simulink model "coeff_bank_simple_test"  (R2021b)
settings: Solver=FixedStepDiscrete  StartTime=0.0  StopTime=stop_time  RelTol=1e-3
values from neighbouring files (symbols this model uses):
  coeff_bitwidth = ul_filter_attribs.coeff_bitwidth    [coeff_bank_simple_testground.m]
  coeff_complex = ul_filter_attribs.complex    [coeff_bank_simple_testground.m]
  coeff_num = ul_filter_attribs.coeff_num    [coeff_bank_simple_testground.m]
libraries: dspsrcs4 x4
settings Model: DataTypeOverride=Off  Creator=torha  LastModifiedBy=torha
settings SolverCC: AlgebraicLoopSolver=TrustRegion
settings OptimizationCC: BlockReduction=off  ConditionallyExecuteInputs=off  DefaultParameterBehavior=Inlined  InheritOutputTypeSmallerThanSingle=on
settings DebuggingCC: AlgebraicLoopMsg=error  SingleTaskRateTransMsg=error  SFMachineParentedDataDiag=warning
settings HardwareCC: ProdBitPerPointer=32  ProdBitPerSizeT=32  ProdBitPerPtrDiffT=32  ProdLargestAtomicFloat=None  ProdIntDivRoundTo=Undefined  ProdEndianess=Unspecified  ProdWordSize=32  ProdHWDeviceType=ASIC/FPGA->ASIC/FPGA  TargetBitPerPointer=64  TargetBitPerSizeT=64  TargetBitPerPtrDiffT=64  TargetLongLongMode=on  TargetIntDivRoundTo=Zero  TargetEndianess=LittleEndian  TargetWordSize=64  TargetHWDeviceType=Custom Processor->MATLAB Host Computer  ProdEqTarget=off

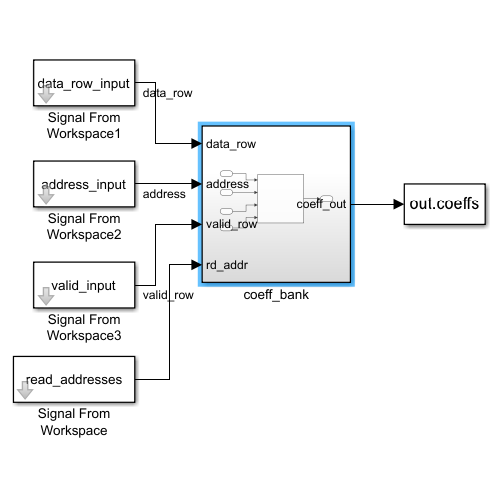
[thumbnail: Simulink's stored preview of the top-level diagram]
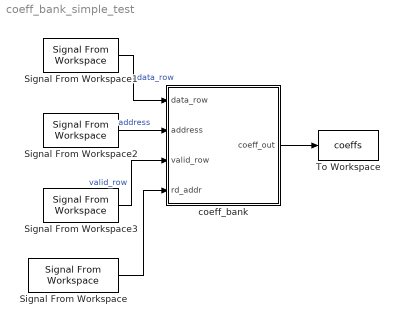
== system coeff_bank_simple_test ==
  Signal From Workspace : dspsrcs4/Signal From Workspace  X=read_addresses  Ts=1  nsamps=1  OutputAfterFinalValue=Setting to zero  ignoreOrWarnInputAndFrameLengths=off  OutputFrames=off
  Signal From Workspace1 : dspsrcs4/Signal From Workspace  X=data_row_input  Ts=1  nsamps=1  OutputAfterFinalValue=Setting to zero  ignoreOrWarnInputAndFrameLengths=off  OutputFrames=off
  Signal From Workspace2 : dspsrcs4/Signal From Workspace  X=address_input  Ts=1  nsamps=1  OutputAfterFinalValue=Setting to zero  ignoreOrWarnInputAndFrameLengths=off  OutputFrames=off
  Signal From Workspace3 : dspsrcs4/Signal From Workspace  X=valid_input  Ts=1  nsamps=1  OutputAfterFinalValue=Setting to zero  ignoreOrWarnInputAndFrameLengths=off  OutputFrames=off
  To Workspace : ToWorkspace  VariableName=coeffs  SampleTime=-1
      settings: Save2DSignal=2-D array (concatenate along first dimension)
  coeff_bank : Subsystem
  wires:
  Signal From Workspace/1 -> coeff_bank/4(rd_addr)
  coeff_bank/1(coeff_out) -> To Workspace/1
  Signal From Workspace2/1 -> coeff_bank/2(address)  "address"
  Signal From Workspace3/1 -> coeff_bank/3(valid_row)  "valid_row"
  Signal From Workspace1/1 -> coeff_bank/1(data_row)  "data_row"

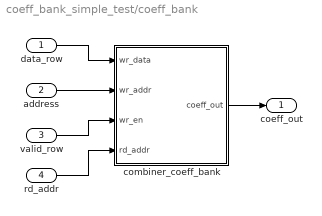
== system coeff_bank_simple_test/coeff_bank ==
  data_row : Inport
  address : Inport  Port=2
  valid_row : Inport  Port=3
  rd_addr : Inport  Port=4
  combiner_coeff_bank : Subsystem  Variant=on  mask{coeff=struct('coeff_num', coeff_num, 'coeff_bitwidth', coeff_bitwidth, 'complex', coeff_complex)}
      mask init:
      | load('constants.mat', 'coeff_ram_bitwidth');
      | last_ram_size = mod(coeff.coeff_bitwidth*coeff.coeff_num*(1+coeff.complex), coeff_ram_bitwidth);
      | if last_ram_size == 0
      |     last_ram_size = coeff_ram_bitwidth;
      | end
      | num_rams = ceil(coeff.coeff_bitwidth*coeff.coeff_num*(1+coeff.complex)/coeff_ram_bitwidth)-1;
  coeff_out : Outport
  wires:
  rd_addr/1 -> combiner_coeff_bank/4(rd_addr)
  data_row/1 -> combiner_coeff_bank/1(wr_data)
  valid_row/1 -> combiner_coeff_bank/3(wr_en)
  address/1 -> combiner_coeff_bank/2(wr_addr)
  combiner_coeff_bank/1(coeff_out) -> coeff_out/1

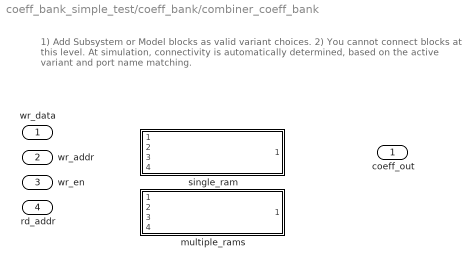
== system coeff_bank_simple_test/coeff_bank/combiner_coeff_bank ==
  note: 1) Add Subsystem or Model blocks as valid variant choices.
      | 2) You cannot connect blocks at this level. At simulation, connectivity is automatically
      | determined, based on the active variant and port name matching.
  wr_data : Inport
  wr_addr : Inport  Port=2
  wr_en : Inport  Port=3
  rd_addr : Inport  Port=4
  multiple_rams : Subsystem  VariantControl=(default)  ReferencedSubsystem=coeff_bank_multiple_rams
  single_ram : Subsystem  VariantControl=num_rams==0  ReferencedSubsystem=coeff_bank_single_ram
  coeff_out : Outport
